simulink model "sampleModel328"  (R2021b)
settings: Solver=VariableStepAuto  StartTime=0.0  StopTime=10.0  RelTol=1e-3
undefined symbols (not defined in the file or in its folder): DiscIntNeverNeededParam, Newton, Raphson
libraries: simulink x2
settings Model: Creator=user  LastModifiedBy=user

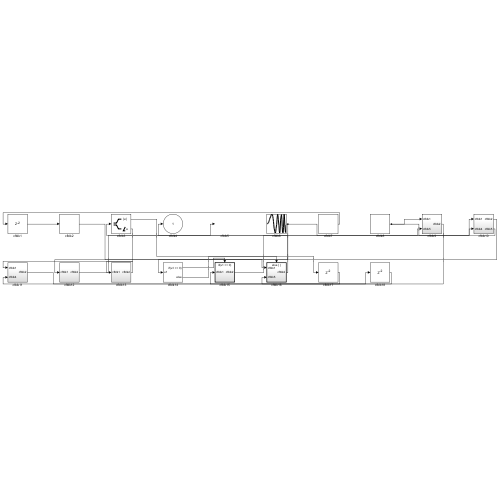
[thumbnail: Simulink's stored preview of the top-level diagram]
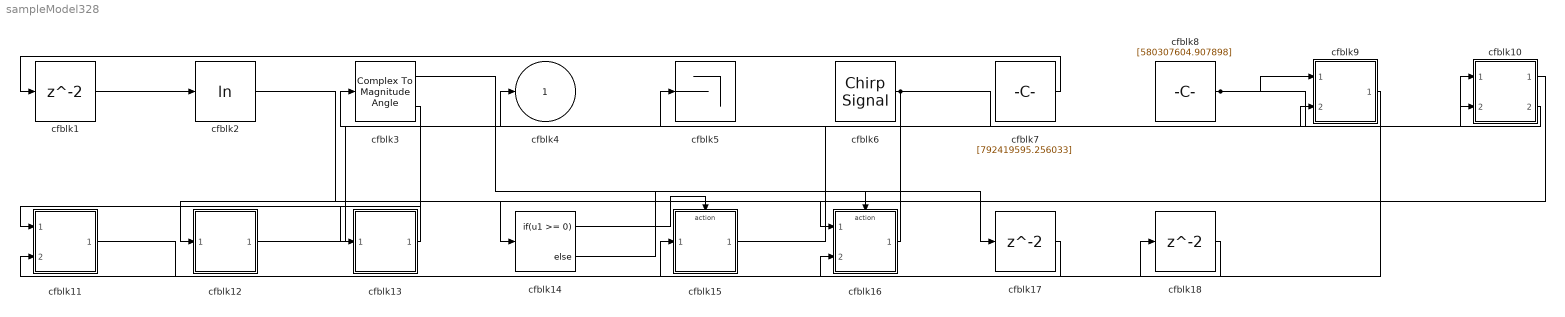
== system sampleModel328 ==
  cfblk1 : Delay  SampleTime=1
  cfblk10 : Subsystem
  cfblk11 : Subsystem
  cfblk12 : Subsystem
  cfblk13 : Subsystem
  cfblk14 : If  IfExpression=u1 >= 0  SampleTime=1
  cfblk15 : Subsystem  TreatAsAtomicUnit=on
  cfblk16 : Subsystem  TreatAsAtomicUnit=on
  cfblk17 : Delay  SampleTime=1
  cfblk18 : Delay  SampleTime=1
  cfblk2 : Math  Operator=log  SaturateOnIntegerOverflow=on
  cfblk3 : ComplexToMagnitudeAngle
  cfblk5 : Terminator
  cfblk6 : simulink/Sources/Chirp Signal  f1=[582127834.262175]  T=[-597744914.863436]  f2=[-553868150.851158]
  cfblk7 : Constant  Value=[792419595.256033]  SampleTime=1
  cfblk8 : Constant  Value=[580307604.907898]  SampleTime=1
  cfblk9 : Subsystem
  cfblk4 : Outport
  wires:
  cfblk16/1(cfblk2) -> cfblk3/1
  cfblk13/1(cfblk2) -> cfblk11/1(cfblk1)
  cfblk12/1(cfblk2) -> cfblk5/1
  cfblk9/1(cfblk2) -> cfblk11/2(cfblk4)
  cfblk3/2 -> cfblk13/1(cfblk1)
  cfblk6/1 -> cfblk14/1, cfblk9/2(cfblk5)
  cfblk1/1 -> cfblk2/1
  cfblk10/1(cfblk2) -> cfblk12/1(cfblk1)
  cfblk10/2(cfblk5) -> cfblk4/1
  cfblk15/1(cfblk2) -> cfblk10/1(cfblk1)
  cfblk2/1 -> cfblk16/1(cfblk1)
  cfblk8/1 -> cfblk10/2(cfblk4), cfblk9/1(cfblk1)
  cfblk7/1 -> cfblk1/1
  cfblk14/1 -> cfblk15/Action
  cfblk14/2 -> cfblk16/Action
  cfblk3/1 -> cfblk17/1
  cfblk17/1 -> cfblk15/1(cfblk1)
  cfblk11/1(cfblk2) -> cfblk18/1
  cfblk18/1 -> cfblk16/2(cfblk5)

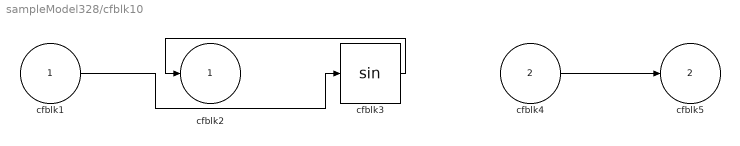
== system sampleModel328/cfblk10 ==
  cfblk1 : Inport
  cfblk4 : Inport  Port=2
  cfblk3 : Trigonometry
  cfblk2 : Outport
  cfblk5 : Outport  Port=2
  wires:
  cfblk3/1 -> cfblk2/1
  cfblk1/1 -> cfblk3/1
  cfblk4/1 -> cfblk5/1

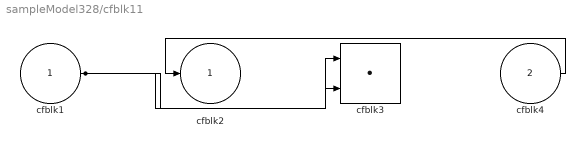
== system sampleModel328/cfblk11 ==
  cfblk1 : Inport
  cfblk4 : Inport  Port=2
  cfblk3 : DotProduct  InputSameDT=on  OutDataTypeStr=Inherit: Inherit via internal rule
  cfblk2 : Outport
  wires:
  cfblk4/1 -> cfblk2/1
  cfblk1/1 -> cfblk3/1, cfblk3/2

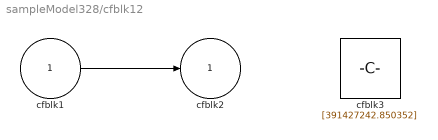
== system sampleModel328/cfblk12 ==
  cfblk1 : Inport
  cfblk3 : Constant  Value=[391427242.850352]  SampleTime=1
  cfblk2 : Outport
  wires:
  cfblk1/1 -> cfblk2/1

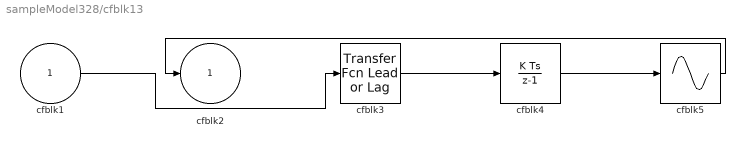
== system sampleModel328/cfblk13 ==
  cfblk1 : Inport
  cfblk3 : simulink/Discrete/Transfer Fcn Lead or Lag  PoleZ=0.95  ZeroZ=0.75  ICPrevOutput=0.0  ICPrevInput=0.0  DoSatur=off
      settings: SourceProductBaseCode=SL
  cfblk4 : DiscreteIntegrator  ICPrevOutput=DiscIntNeverNeededParam  ICPrevScaledInput=DiscIntNeverNeededParam
  cfblk5 : Sin  TimeSource=Use external signal  SampleTime=0
  cfblk2 : Outport
  wires:
  cfblk4/1 -> cfblk5/1
  cfblk5/1 -> cfblk2/1
  cfblk3/1 -> cfblk4/1
  cfblk1/1 -> cfblk3/1

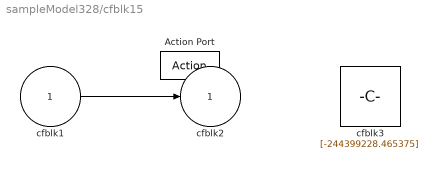
== system sampleModel328/cfblk15 ==
  cfblk1 : Inport
  Action Port : ActionPort  ActionPortLabel=if(u1 >= 0)
  cfblk3 : Constant  Value=[-244399228.465375]  SampleTime=1
  cfblk2 : Outport
  wires:
  cfblk1/1 -> cfblk2/1

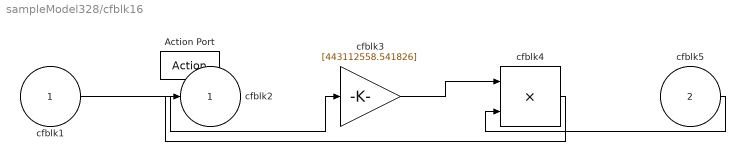
== system sampleModel328/cfblk16 ==
  cfblk1 : Inport
  cfblk5 : Inport  Port=2
  Action Port : ActionPort  ActionPortLabel=else
  cfblk3 : Gain  Gain=[443112558.541826]
  cfblk4 : Product
  cfblk2 : Outport
  wires:
  cfblk1/1 -> cfblk3/1
  cfblk3/1 -> cfblk4/1
  cfblk4/1 -> cfblk2/1
  cfblk5/1 -> cfblk4/2

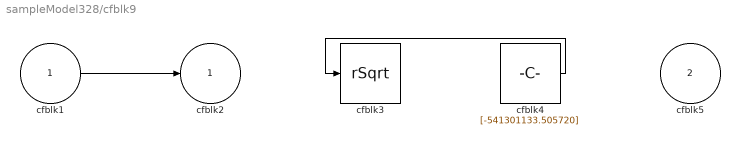
== system sampleModel328/cfblk9 ==
  cfblk1 : Inport
  cfblk5 : Inport  Port=2
  cfblk3 : Sqrt  Operator=rSqrt  AlgorithmType=Newton-Raphson  SaturateOnIntegerOverflow=on
  cfblk4 : Constant  Value=[-541301133.505720]  SampleTime=1
  cfblk2 : Outport
  wires:
  cfblk1/1 -> cfblk2/1
  cfblk4/1 -> cfblk3/1
